simulink model "building_PHPP_v1"  (R2018b)
settings: Solver=ode23s  StartTime=-building.preruntime+8760*3600  StopTime=building.runtime+8760*3600  EnableMultiTasking=on
StartFcn:
  | tic
StopFcn:
  | toc
values from neighbouring files (symbols this model uses):
  A = 7*10*2    (= 140)    [theta_ground_v1.m]    (also in xlswrite1.m = num2cell(data))
  B = A/(0.5 * P)    (= 8.23529411765)    [theta_ground_v1.m]
  building = obj    [BUILDING.m]    (also in create_building_automatic.m = building.save(); ini_building_automatic.m = building.add_variant_hvac(building.variant_hvac, hvac); load_building_automatic.m = building.save())
  C = zeros(1,length(d)+1)    [CONSTRUCTION.m]    (also in DOOR.m = [0 0 0]; WALL.m = [0 0 0]; WINDOW.m = [0 0 0])
  cp = str2num(value)    [CONSTRUCTION.m]
  p = [timevec_weather weather(:,12)]    [BOUNDARY.m]    (also in WEATHER.m = 0; init_carnotUIBK.m = cell2mat(carnotUIBKpaths(i,2)))
  rho = str2num(value)    [CONSTRUCTION.m]    (also in theta_ground_v1.m = 2000)
undefined symbols (not defined in the file or in its folder): Dd, Dreifach, get_building, Qdot_C, Qdot_C_energy, Qdot_H, Qdot_H_energy, Qdot_I_electricity, Qdot_I_electricity_energy, Qdot_I_light, Qdot_I_light_energy, Qdot_I_person, Qdot_I_person_energy, Qdot_S, Qdot_S_energy, Qdot_T_ground, Qdot_T_ground_energy, Qdot_T_neighbour, Qdot_T_neighbour_energy, Qdot_T_opaque, Qdot_T_opaque_energy, Qdot_T_window, Qdot_T_window_energy, Qdot_V_infiltration, Qdot_V_infiltration_energy, Qdot_V_mech, Qdot_V_mech_energy, Qdot_V_window, Qdot_V_window_energy, Tc, Tr, Ts, Wärmeschutzglas, x_CO2, x_H2O, x_VOC
libraries: carnotUIBK x1874, carnot x5, simulink x3
(part 34 of 34)

== system building_PHPP_v1/DATALOGGER/logger_BDB/z7/Subsystem1 ==
  In1 : Inport
  Integrator1 : Integrator
  Ws->kWh : Gain  Gain=1/3600/1000
  Out1 : Outport
  wires:
  In1/1 -> Integrator1/1
  Integrator1/1 -> Ws->kWh/1
  Ws->kWh/1 -> Out1/1

== system building_PHPP_v1/DATALOGGER/logger_BDB/z7/Subsystem10 ==
  In1 : Inport
  Integrator1 : Integrator
  Ws->kWh : Gain  Gain=1/3600/1000
  Out1 : Outport
  wires:
  Ws->kWh/1 -> Out1/1
  Integrator1/1 -> Ws->kWh/1
  In1/1 -> Integrator1/1

== system building_PHPP_v1/DATALOGGER/logger_BDB/z7/Subsystem11 ==
  In1 : Inport
  Integrator1 : Integrator
  Ws->kWh : Gain  Gain=1/3600/1000
  Out1 : Outport
  wires:
  In1/1 -> Integrator1/1
  Integrator1/1 -> Ws->kWh/1
  Ws->kWh/1 -> Out1/1

== system building_PHPP_v1/DATALOGGER/logger_BDB/z7/Subsystem12 ==
  In1 : Inport
  Integrator1 : Integrator
  Ws->kWh : Gain  Gain=1/3600/1000
  Out1 : Outport
  wires:
  Ws->kWh/1 -> Out1/1
  Integrator1/1 -> Ws->kWh/1
  In1/1 -> Integrator1/1

== system building_PHPP_v1/DATALOGGER/logger_BDB/z7/Subsystem2 ==
  In1 : Inport
  Integrator1 : Integrator
  Ws->kWh : Gain  Gain=1/3600/1000
  Out1 : Outport
  wires:
  Ws->kWh/1 -> Out1/1
  Integrator1/1 -> Ws->kWh/1
  In1/1 -> Integrator1/1

== system building_PHPP_v1/DATALOGGER/logger_BDB/z7/Subsystem3 ==
  In1 : Inport
  Integrator1 : Integrator
  Ws->kWh : Gain  Gain=1/3600/1000
  Out1 : Outport
  wires:
  In1/1 -> Integrator1/1
  Integrator1/1 -> Ws->kWh/1
  Ws->kWh/1 -> Out1/1

== system building_PHPP_v1/DATALOGGER/logger_BDB/z7/Subsystem4 ==
  In1 : Inport
  Integrator1 : Integrator
  Ws->kWh : Gain  Gain=1/3600/1000
  Out1 : Outport
  wires:
  Ws->kWh/1 -> Out1/1
  Integrator1/1 -> Ws->kWh/1
  In1/1 -> Integrator1/1

== system building_PHPP_v1/DATALOGGER/logger_BDB/z7/Subsystem5 ==
  In1 : Inport
  Integrator1 : Integrator
  Ws->kWh : Gain  Gain=1/3600/1000
  Out1 : Outport
  wires:
  In1/1 -> Integrator1/1
  Integrator1/1 -> Ws->kWh/1
  Ws->kWh/1 -> Out1/1

== system building_PHPP_v1/DATALOGGER/logger_BDB/z7/Subsystem6 ==
  In1 : Inport
  Integrator1 : Integrator
  Ws->kWh : Gain  Gain=1/3600/1000
  Out1 : Outport
  wires:
  Ws->kWh/1 -> Out1/1
  Integrator1/1 -> Ws->kWh/1
  In1/1 -> Integrator1/1

== system building_PHPP_v1/DATALOGGER/logger_BDB/z7/Subsystem7 ==
  In1 : Inport
  Integrator1 : Integrator
  Ws->kWh : Gain  Gain=1/3600/1000
  Out1 : Outport
  wires:
  In1/1 -> Integrator1/1
  Integrator1/1 -> Ws->kWh/1
  Ws->kWh/1 -> Out1/1

== system building_PHPP_v1/DATALOGGER/logger_BDB/z7/Subsystem8 ==
  In1 : Inport
  Integrator1 : Integrator
  Ws->kWh : Gain  Gain=1/3600/1000
  Out1 : Outport
  wires:
  Ws->kWh/1 -> Out1/1
  Integrator1/1 -> Ws->kWh/1
  In1/1 -> Integrator1/1

== system building_PHPP_v1/DATALOGGER/logger_BDB/z7/Subsystem9 ==
  In1 : Inport
  Integrator1 : Integrator
  Ws->kWh : Gain  Gain=1/3600/1000
  Out1 : Outport
  wires:
  In1/1 -> Integrator1/1
  Integrator1/1 -> Ws->kWh/1
  Ws->kWh/1 -> Out1/1

== system building_PHPP_v1/DATALOGGER/logger_BDB/z8/Subsystem ==
  In1 : Inport
  Integrator1 : Integrator
  Ws->kWh : Gain  Gain=1/3600/1000
  Out1 : Outport
  wires:
  In1/1 -> Integrator1/1
  Integrator1/1 -> Ws->kWh/1
  Ws->kWh/1 -> Out1/1

== system building_PHPP_v1/DATALOGGER/logger_BDB/z8/Subsystem1 ==
  In1 : Inport
  Integrator1 : Integrator
  Ws->kWh : Gain  Gain=1/3600/1000
  Out1 : Outport
  wires:
  Ws->kWh/1 -> Out1/1
  Integrator1/1 -> Ws->kWh/1
  In1/1 -> Integrator1/1

== system building_PHPP_v1/DATALOGGER/logger_BDB/z8/Subsystem10 ==
  In1 : Inport
  Integrator1 : Integrator
  Ws->kWh : Gain  Gain=1/3600/1000
  Out1 : Outport
  wires:
  In1/1 -> Integrator1/1
  Integrator1/1 -> Ws->kWh/1
  Ws->kWh/1 -> Out1/1

== system building_PHPP_v1/DATALOGGER/logger_BDB/z8/Subsystem11 ==
  In1 : Inport
  Integrator1 : Integrator
  Ws->kWh : Gain  Gain=1/3600/1000
  Out1 : Outport
  wires:
  Ws->kWh/1 -> Out1/1
  Integrator1/1 -> Ws->kWh/1
  In1/1 -> Integrator1/1

== system building_PHPP_v1/DATALOGGER/logger_BDB/z8/Subsystem12 ==
  In1 : Inport
  Integrator1 : Integrator
  Ws->kWh : Gain  Gain=1/3600/1000
  Out1 : Outport
  wires:
  In1/1 -> Integrator1/1
  Integrator1/1 -> Ws->kWh/1
  Ws->kWh/1 -> Out1/1

== system building_PHPP_v1/DATALOGGER/logger_BDB/z8/Subsystem2 ==
  In1 : Inport
  Integrator1 : Integrator
  Ws->kWh : Gain  Gain=1/3600/1000
  Out1 : Outport
  wires:
  In1/1 -> Integrator1/1
  Integrator1/1 -> Ws->kWh/1
  Ws->kWh/1 -> Out1/1

== system building_PHPP_v1/DATALOGGER/logger_BDB/z8/Subsystem3 ==
  In1 : Inport
  Integrator1 : Integrator
  Ws->kWh : Gain  Gain=1/3600/1000
  Out1 : Outport
  wires:
  Ws->kWh/1 -> Out1/1
  Integrator1/1 -> Ws->kWh/1
  In1/1 -> Integrator1/1

== system building_PHPP_v1/DATALOGGER/logger_BDB/z8/Subsystem4 ==
  In1 : Inport
  Integrator1 : Integrator
  Ws->kWh : Gain  Gain=1/3600/1000
  Out1 : Outport
  wires:
  In1/1 -> Integrator1/1
  Integrator1/1 -> Ws->kWh/1
  Ws->kWh/1 -> Out1/1

== system building_PHPP_v1/DATALOGGER/logger_BDB/z8/Subsystem5 ==
  In1 : Inport
  Integrator1 : Integrator
  Ws->kWh : Gain  Gain=1/3600/1000
  Out1 : Outport
  wires:
  Ws->kWh/1 -> Out1/1
  Integrator1/1 -> Ws->kWh/1
  In1/1 -> Integrator1/1

== system building_PHPP_v1/DATALOGGER/logger_BDB/z8/Subsystem6 ==
  In1 : Inport
  Integrator1 : Integrator
  Ws->kWh : Gain  Gain=1/3600/1000
  Out1 : Outport
  wires:
  In1/1 -> Integrator1/1
  Integrator1/1 -> Ws->kWh/1
  Ws->kWh/1 -> Out1/1

== system building_PHPP_v1/DATALOGGER/logger_BDB/z8/Subsystem7 ==
  In1 : Inport
  Integrator1 : Integrator
  Ws->kWh : Gain  Gain=1/3600/1000
  Out1 : Outport
  wires:
  Ws->kWh/1 -> Out1/1
  Integrator1/1 -> Ws->kWh/1
  In1/1 -> Integrator1/1

== system building_PHPP_v1/DATALOGGER/logger_BDB/z8/Subsystem8 ==
  In1 : Inport
  Integrator1 : Integrator
  Ws->kWh : Gain  Gain=1/3600/1000
  Out1 : Outport
  wires:
  In1/1 -> Integrator1/1
  Integrator1/1 -> Ws->kWh/1
  Ws->kWh/1 -> Out1/1

== system building_PHPP_v1/DATALOGGER/logger_BDB/z8/Subsystem9 ==
  In1 : Inport
  Integrator1 : Integrator
  Ws->kWh : Gain  Gain=1/3600/1000
  Out1 : Outport
  wires:
  Ws->kWh/1 -> Out1/1
  Integrator1/1 -> Ws->kWh/1
  In1/1 -> Integrator1/1

== system building_PHPP_v1/DATALOGGER/logger_BDB/z9/Subsystem ==
  In1 : Inport
  Integrator1 : Integrator
  Ws->kWh : Gain  Gain=1/3600/1000
  Out1 : Outport
  wires:
  Ws->kWh/1 -> Out1/1
  Integrator1/1 -> Ws->kWh/1
  In1/1 -> Integrator1/1

== system building_PHPP_v1/DATALOGGER/logger_BDB/z9/Subsystem1 ==
  In1 : Inport
  Integrator1 : Integrator
  Ws->kWh : Gain  Gain=1/3600/1000
  Out1 : Outport
  wires:
  In1/1 -> Integrator1/1
  Integrator1/1 -> Ws->kWh/1
  Ws->kWh/1 -> Out1/1

== system building_PHPP_v1/DATALOGGER/logger_BDB/z9/Subsystem10 ==
  In1 : Inport
  Integrator1 : Integrator
  Ws->kWh : Gain  Gain=1/3600/1000
  Out1 : Outport
  wires:
  Ws->kWh/1 -> Out1/1
  Integrator1/1 -> Ws->kWh/1
  In1/1 -> Integrator1/1

== system building_PHPP_v1/DATALOGGER/logger_BDB/z9/Subsystem11 ==
  In1 : Inport
  Integrator1 : Integrator
  Ws->kWh : Gain  Gain=1/3600/1000
  Out1 : Outport
  wires:
  In1/1 -> Integrator1/1
  Integrator1/1 -> Ws->kWh/1
  Ws->kWh/1 -> Out1/1

== system building_PHPP_v1/DATALOGGER/logger_BDB/z9/Subsystem12 ==
  In1 : Inport
  Integrator1 : Integrator
  Ws->kWh : Gain  Gain=1/3600/1000
  Out1 : Outport
  wires:
  Ws->kWh/1 -> Out1/1
  Integrator1/1 -> Ws->kWh/1
  In1/1 -> Integrator1/1

== system building_PHPP_v1/DATALOGGER/logger_BDB/z9/Subsystem2 ==
  In1 : Inport
  Integrator1 : Integrator
  Ws->kWh : Gain  Gain=1/3600/1000
  Out1 : Outport
  wires:
  Ws->kWh/1 -> Out1/1
  Integrator1/1 -> Ws->kWh/1
  In1/1 -> Integrator1/1

== system building_PHPP_v1/DATALOGGER/logger_BDB/z9/Subsystem3 ==
  In1 : Inport
  Integrator1 : Integrator
  Ws->kWh : Gain  Gain=1/3600/1000
  Out1 : Outport
  wires:
  In1/1 -> Integrator1/1
  Integrator1/1 -> Ws->kWh/1
  Ws->kWh/1 -> Out1/1

== system building_PHPP_v1/DATALOGGER/logger_BDB/z9/Subsystem4 ==
  In1 : Inport
  Integrator1 : Integrator
  Ws->kWh : Gain  Gain=1/3600/1000
  Out1 : Outport
  wires:
  Ws->kWh/1 -> Out1/1
  Integrator1/1 -> Ws->kWh/1
  In1/1 -> Integrator1/1

== system building_PHPP_v1/DATALOGGER/logger_BDB/z9/Subsystem5 ==
  In1 : Inport
  Integrator1 : Integrator
  Ws->kWh : Gain  Gain=1/3600/1000
  Out1 : Outport
  wires:
  In1/1 -> Integrator1/1
  Integrator1/1 -> Ws->kWh/1
  Ws->kWh/1 -> Out1/1

== system building_PHPP_v1/DATALOGGER/logger_BDB/z9/Subsystem6 ==
  In1 : Inport
  Integrator1 : Integrator
  Ws->kWh : Gain  Gain=1/3600/1000
  Out1 : Outport
  wires:
  Ws->kWh/1 -> Out1/1
  Integrator1/1 -> Ws->kWh/1
  In1/1 -> Integrator1/1

== system building_PHPP_v1/DATALOGGER/logger_BDB/z9/Subsystem7 ==
  In1 : Inport
  Integrator1 : Integrator
  Ws->kWh : Gain  Gain=1/3600/1000
  Out1 : Outport
  wires:
  In1/1 -> Integrator1/1
  Integrator1/1 -> Ws->kWh/1
  Ws->kWh/1 -> Out1/1

== system building_PHPP_v1/DATALOGGER/logger_BDB/z9/Subsystem8 ==
  In1 : Inport
  Integrator1 : Integrator
  Ws->kWh : Gain  Gain=1/3600/1000
  Out1 : Outport
  wires:
  Ws->kWh/1 -> Out1/1
  Integrator1/1 -> Ws->kWh/1
  In1/1 -> Integrator1/1

== system building_PHPP_v1/DATALOGGER/logger_BDB/z9/Subsystem9 ==
  In1 : Inport
  Integrator1 : Integrator
  Ws->kWh : Gain  Gain=1/3600/1000
  Out1 : Outport
  wires:
  In1/1 -> Integrator1/1
  Integrator1/1 -> Ws->kWh/1
  Ws->kWh/1 -> Out1/1
